simulink model "Lag_Graphical"  (R2022b)
settings: Solver=VariableStepAuto  StartTime=0.0  StopTime=15  RelTol=1e-3
libraries: simulink x3
settings Model: Creator=amirz  LastModifiedBy=amirz

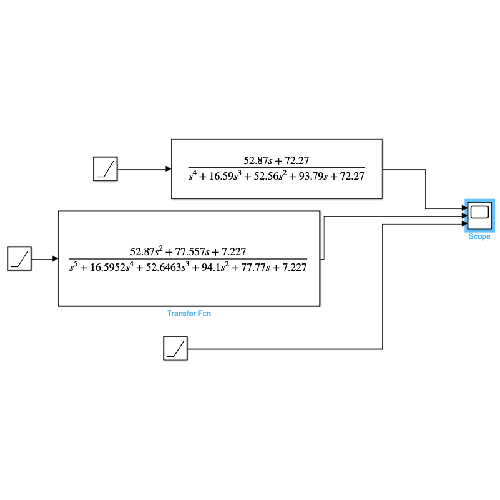
[thumbnail: Simulink's stored preview of the top-level diagram]
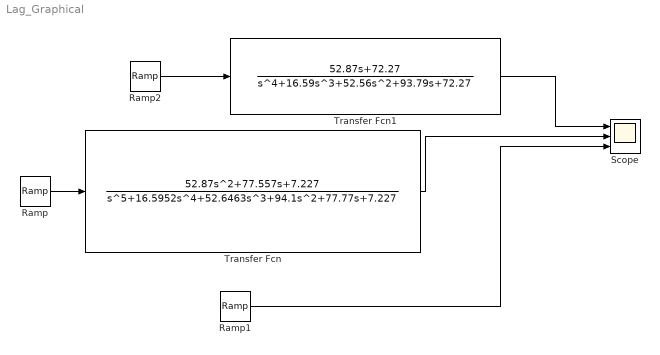
== system Lag_Graphical ==
  Ramp : simulink/Sources/Ramp  slope=1  start=0  InitialOutput=0
  Ramp1 : simulink/Sources/Ramp  slope=1  start=0  InitialOutput=0
  Ramp2 : simulink/Sources/Ramp  slope=1  start=0  InitialOutput=0
  Scope : Scope  NumInputPorts=3
  Transfer Fcn : TransferFcn  Numerator=[52.87 77.557 7.227]  Denominator=[1 16.5952 52.6463 94.1 77.77 7.227]
  Transfer Fcn1 : TransferFcn  Numerator=[52.87 72.27]  Denominator=[1 16.59 52.56 93.79 72.27]
  wires:
  Ramp/1 -> Transfer Fcn/1
  Transfer Fcn/1 -> Scope/2
  Ramp1/1 -> Scope/3
  Ramp2/1 -> Transfer Fcn1/1
  Transfer Fcn1/1 -> Scope/1
